simulink model "rezervorul"  (R2022b)
settings: Solver=VariableStepAuto  StartTime=0.0  StopTime=10.0  RelTol=1e-3
settings Model: Creator=Ruxandra  LastModifiedBy=Ruxandra

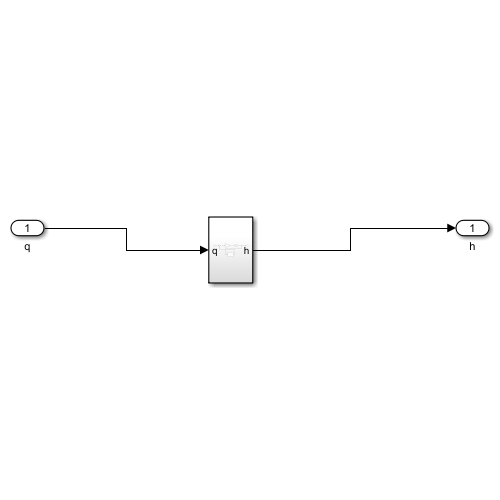
[thumbnail: Simulink's stored preview of the top-level diagram]
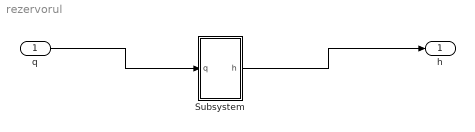
== system rezervorul ==
  q : Inport
  Subsystem : Subsystem
  h : Outport
  wires:
  q/1 -> Subsystem/1(q)
  Subsystem/1(h) -> h/1

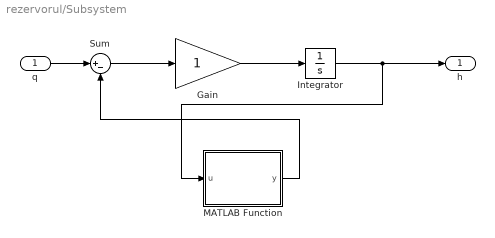
== system rezervorul/Subsystem ==
  q : Inport
  Gain : Gain
  Integrator : Integrator
  MATLAB Function : MATLAB Function  TreatAsAtomicUnit=on
  Sum : Sum  Inputs=|+-
  h : Outport
  wires:
  Integrator/1 -> h/1, MATLAB Function/1(u)
  q/1 -> Sum/1
  Gain/1 -> Integrator/1
  MATLAB Function/1(y) -> Sum/2
  Sum/1 -> Gain/1

== matlab function rezervorul/Subsystem/MATLAB Function ==
  data: u input; y output
function y = sqrt(u)

y = sqrt(u)*9;
